simulink model "turbine_and_control_simulation"  (R2019a)
settings: Solver=FixedStepAuto  StartTime=0.0  StopTime=3600  FixedStep=0.1  RelTol=1e-3
values from neighbouring files (symbols this model uses):
  V = zeros(3600*length(vel),1)    [code_for_control.m]
libraries: simulink x1, powerlib x1
settings Model: Creator=artur  LastModifiedBy=artur

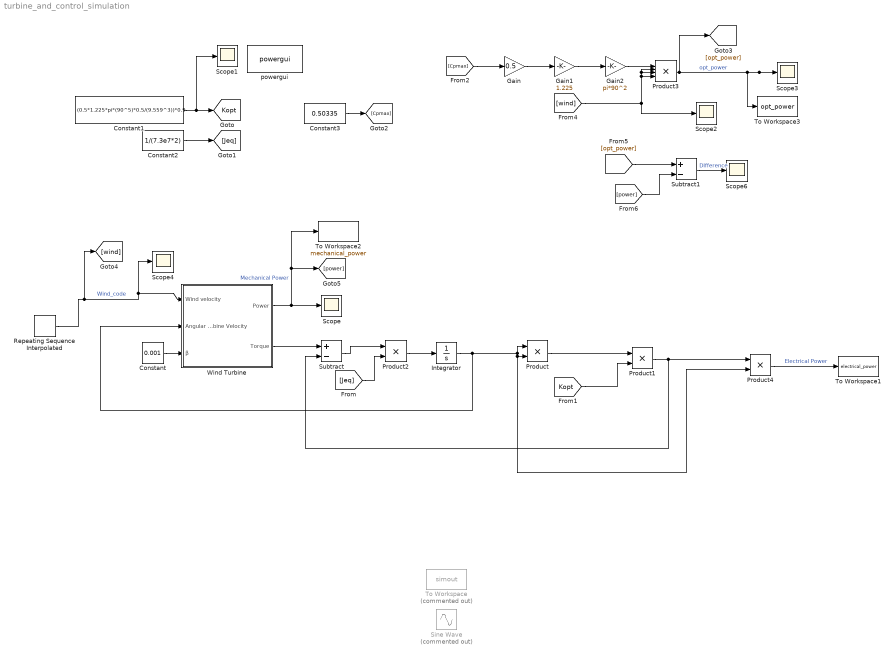
== system turbine_and_control_simulation ==
  Constant : Constant  Value=0.001
  Constant1 : Constant  Value=(0.5*1.225*pi*(90^5)*0.5/(9.559^3))*0.9
  Constant2 : Constant  Value=1/(7.3e7*2)
  Constant3 : Constant  Value=0.50335
  Gain : Gain  Gain=0.5
  Gain1 : Gain  Gain=1.225
  Gain2 : Gain  Gain=pi*90^2
  Integrator : Integrator  InitialCondition=6.5043*V(1)/90
  Product{,1..2,4} (4 alike) : Product
  Product3 : Product  Inputs=4
  Repeating Sequence Interpolated : simulink/Sources/Repeating Sequence Interpolated  OutValues=V  TimeValues=1:length(V).'  LookUpMeth=Interpolation-Use End Values  tsamp=0.1  OutMin=[]  OutMax=[]  OutDataTypeStr=double  OutputDataTypeScalingMode=double  OutDataType=fixdt(0,8)  OutScaling=2^-10
  Scope{,1..4,6} (6 alike) : Scope
  Sine Wave : Sin  Commented=on  Amplitude=3  Bias=8  Frequency=2*pi/200  SampleTime=0
  Subtract : Sum  Inputs=+-
  Subtract1 : Sum  Inputs=+-
  To Workspace : ToWorkspace  Commented=on  VariableName=simout  SaveFormat=Timeseries  SampleTime=-1
  To Workspace1 : ToWorkspace  VariableName=electrical_power  SampleTime=1
  To Workspace2 : ToWorkspace  VariableName=mechanical_power  SampleTime=1
  To Workspace3 : ToWorkspace  VariableName=opt_power  SampleTime=1
  "Wind Turbine " : Subsystem
  powergui : powerlib/powergui  Priority=1  SimulationMode=Continuous  SampleTime=0.001  frequency=60  Iterations=50  frequencyindice=60  Pbase=100e6  ErrMax=1e-4  UnitsV=kV  UnitsW=MW  buscounter=0  FunctionMessages=off  echomessages=off  EnableUseOfTLC=off  CurrentSourceSwitches=off  DisableSnubberDevices=off  DisableRonSwitches=off  DisableVfSwitches=off  DisplayEquations=off  AutomaticDiscreteSolvers=off  SolverType=Tustin/Backward Euler (TBE)  Interpol=off  ExternalGateDelay=off  methode=off  Ts=100  x0status=blocks  SPID=on  SwTol=0  HookPort=off  NonlinearTolerance=0  nMaxIteration=15  ContinueOnMaxIteration=off  RestoreLinks=warning  ResistiveCurrentMeasurement=off  Frange=[0:2:500]  Ylog=off  Xlog=on  ShowGrid=off  save=off  variable=ZData  structure=0  ZoomFFT=off  StartTime=0.0  cycles=1  DisplayStyle=1  fundamental=60  FreqAxis=off  MaxFrequency=1000  frequencyindicesteady=1  RmsSteady=1  display=off
      settings: SourceProductName=Simscape Electrical
  tag scope: Kopt=global
  wires:
  Repeating Sequence Interpolated/1 -> Scope4/1, "Wind Turbine "/1("Wind velocity "), [wind]  "Wind_code"
  Constant/1 -> "Wind Turbine "/3("β ")
  "Wind Turbine "/1("Power ") -> To Workspace2/1, [power], Scope/1  "Mechanical Power"
  "Wind Turbine "/2("Torque ") -> Subtract/1
  Subtract/1 -> Product2/1
  Product2/1 -> Integrator/1
  Integrator/1 -> Product/2, Product4/2, Product/1, "Wind Turbine "/2("Angular Turbine Velocity ")
  Product/1 -> Product1/1
  Product1/1 -> Product4/1, Subtract/2
  [Jeq] -> Product2/2
  Constant1/1 -> Scope1/1, [Kopt]
  Constant2/1 -> [Jeq]
  [Kopt] -> Product1/2
  Constant3/1 -> [Cpmax]
  [Cpmax] -> Gain/1
  Gain/1 -> Gain1/1
  Gain1/1 -> Gain2/1
  Gain2/1 -> Product3/1
  [wind] -> Scope2/1, Product3/3, Product3/2, Product3/4
  Product3/1 -> [opt_power], To Workspace3/1, Scope3/1  "opt_power"
  [opt_power] -> Subtract1/1
  [power] -> Subtract1/2
  Subtract1/1 -> Scope6/1  "DIfference"
  Product4/1 -> To Workspace1/1  "Electrical Power"

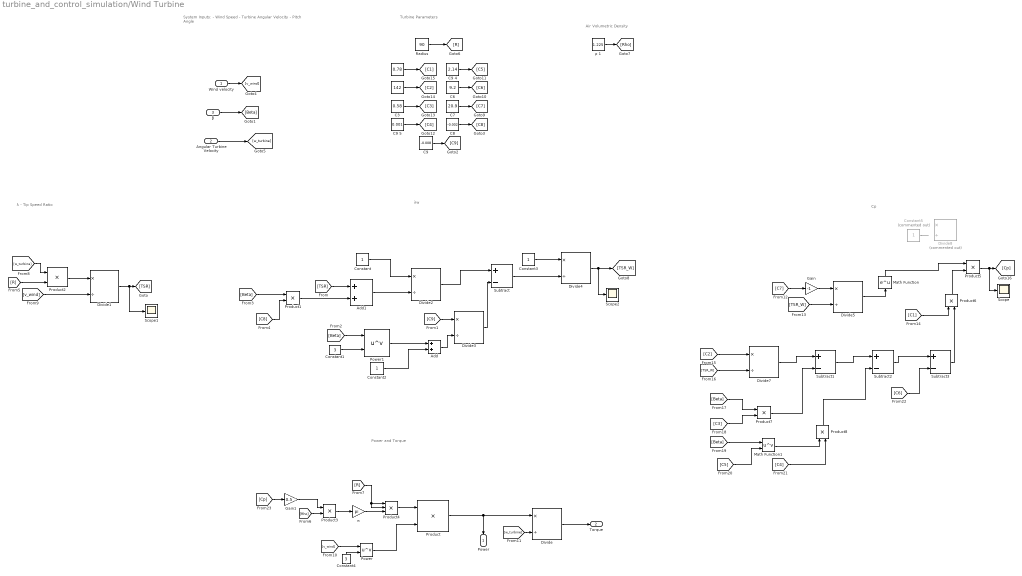
== system turbine_and_control_simulation/Wind Turbine  ==
  note: Power and Torque
  note: λw
  note: λ - Tip Speed Ratio
  note: System Inputs:
      | - Wind Speed
      | - Turbine Angular Velocity
      | - Pitch Angle
  note: Turbine Parameters
  note: Air Volumetric Density
  note: Cp
  "Wind velocity " : Inport
  "Angular Turbine Velocity " : Inport  Port=2
  "β " : Inport  Port=3
  " " : Constant  Value=142
  " " : Constant  Value=0.78
  Add : Sum
  Add1 : Sum
  "C3 " : Constant  Value=0.58
  "C6 " : Constant  Value=9.2
  "C7 " : Constant  Value=20.9
  "C8 " : Constant  Value=-0.002
  "C9 " : Constant  Value=-0.008
  C9 4 : Constant  Value=2.14
  C9 5 : Constant  Value=0.001
  Constant : Constant
  Constant1 : Constant  Value=3
  Constant2 : Constant
  Constant3 : Constant
  Constant4 : Constant  Value=3
  Constant5 : Constant  Commented=on
  Divide{,1..5,7} (7 alike) : Product  Inputs=*/
  Divide8 : Product  Commented=on  Inputs=*/
  Gain : Gain  Gain=-1
  Gain1 : Gain  Gain=0.5
  Math Function : Math  SaturateOnIntegerOverflow=on
  Math Function1 : Math  Operator=pow  SaturateOnIntegerOverflow=on
  Power : Math  Operator=pow  SaturateOnIntegerOverflow=on
  Power1 : Math  Operator=pow  SaturateOnIntegerOverflow=on
  Product{,1..3,5..8} (8 alike) : Product
  Product4 : Product  Inputs=3
  "Radius " : Constant  Value=90
  Scope : Scope
  Scope1 : Scope
  Scope2 : Scope
  Subtract{,1..3} (4 alike) : Sum  Inputs=+-
  π : Gain  Gain=pi
  ρ 1 : Constant  Value=1.225
  "Power " : Outport
  "Torque " : Outport  Port=2
  wires:
  [Beta] -> Power1/1
  [C1] -> Product6/1
  C9 4/1 -> [C5]
  [w_turbine] -> Product2/1
  Product7/1 -> Subtract1/2
  "C7 "/1 -> [C7]
  [v_wind] -> Power/1
  [C6] -> Subtract3/2
  "C8 "/1 -> [C8]
  [v_wind] -> Divide1/2
  π/1 -> Product4/3
  [C2] -> Divide7/1
  [TSR_W] -> Divide7/2
  "C9 "/1 -> [C9]
  Subtract/1 -> Divide4/2
  [TSR] -> Add1/1
  [R] -> Product2/2
  [C5] -> Math Function1/2
  Math Function1/1 -> Product8/1
  Gain/1 -> Divide5/1
  Product4/1 -> Product/1
  Divide3/1 -> Subtract/2
  Divide2/1 -> Subtract/1
  "C3 "/1 -> [C3]
  Add/1 -> Divide3/2
  Power1/1 -> Add/1
  ρ 1/1 -> [Rho]
  Constant3/1 -> Divide4/1
  [Rho] -> Product3/2
  Product1/1 -> Add1/2
  Constant/1 -> Divide2/1
  Product2/1 -> Divide1/1
  Product3/1 -> π/1
  Divide/1 -> "Torque "/1
  [C9] -> Divide3/1
  [R] -> Product4/2, Product4/1
  Product/1 -> "Power "/1, Divide/1
  Add1/1 -> Divide2/2
  Constant1/1 -> Power1/2
  [C3] -> Product7/2
  "Wind velocity "/1 -> [v_wind]
  Divide7/1 -> Subtract1/1
  Constant2/1 -> Add/2
  Divide1/1 -> Scope1/1, [TSR]
  Product8/1 -> Subtract2/2
  Constant4/1 -> Power/2
  [C7] -> Gain/1
  Constant5/1 -> ?
  Subtract2/1 -> Subtract3/1
  Gain1/1 -> Product3/1
  " "/1 -> [C1]
  Power/1 -> Product/2
  Subtract1/1 -> Subtract2/1
  Product6/1 -> Product5/2
  Divide4/1 -> Scope2/1, [TSR_W]
  [C4] -> Product8/2
  Subtract3/1 -> Product6/2
  "C6 "/1 -> [C6]
  Product5/1 -> Scope/1, [Cp]
  [Beta] -> Product1/1
  [C8] -> Product1/2
  "Radius "/1 -> [R]
  Divide5/1 -> Math Function/1
  [Cp] -> Gain1/1
  [w_turbine] -> Divide/2
  Math Function/1 -> Product5/1
  [Beta] -> Product7/1
  [Beta] -> Math Function1/1
  [TSR_W] -> Divide5/2
  "β "/1 -> [Beta]
  C9 5/1 -> [C4]
  " "/1 -> [C2]
  "Angular Turbine Velocity "/1 -> [w_turbine]
